simulink model "UAV"  (R2025b)
settings: Solver=ode3  StartTime=0.0  StopTime=inf  FixedStep=Sim.Ts_fisica  RelTol=1e-3
PostLoadFcn:
  | Init
InitFcn:
  | Init
model workspace (MAT data in the model file):
  Mass = 1
undefined symbols (not defined in the file): DiscIntNeverNeededParam, Drone, DWORK0, DWORK1, DWORK10, DWORK11, DWORK12, DWORK13, DWORK14, DWORK15, DWORK16, DWORK17, DWORK18, DWORK19, DWORK2, DWORK20, DWORK21, DWORK22, DWORK23, DWORK24, DWORK3, DWORK4, DWORK5, DWORK6, DWORK7, DWORK8, DWORK9, F, Light, MIL, Sim
libraries: simulink x35, slpidlib x11, vrlib x4, aerolibwind2 x2, sim3dlib x2, uavsim3dlib x2
(part 3 of 8)

== system UAV/untitledPanel1 ==
  Knob : KnobBlock  Tag=HiddenForWebPanel  PanelInfo="{\"height\":258,\"left\":614,\"panelId\":\"panelId-871049d7-78ac-4d7f-b4f9-794c823d572e\",\"top\":77,\"type\":\"panelChild\",\"version\":\"2019b\",\"width\":247,\"zIndex\":1500002}"  LabelPosition=Hide
  Knob1 : KnobBlock  Tag=HiddenForWebPanel  PanelInfo="{\"height\":258,\"left\":52,\"panelId\":\"panelId-871049d7-78ac-4d7f-b4f9-794c823d572e\",\"top\":77,\"type\":\"panelChild\",\"version\":\"2019b\",\"width\":247,\"zIndex\":1500006}"  LabelPosition=Hide  ScaleMax=15  TickInterval=1
  Knob2 : KnobBlock  Tag=HiddenForWebPanel  PanelInfo="{\"height\":258,\"left\":333,\"panelId\":\"panelId-871049d7-78ac-4d7f-b4f9-794c823d572e\",\"top\":77,\"type\":\"panelChild\",\"version\":\"2019b\",\"width\":247,\"zIndex\":1500004}"  LabelPosition=Hide  ScaleMax=360  TickInterval=45
  panelInfo : PanelWebBlock  Tag=HiddenForWebPanel  PanelInfo="{\"compacted\":false,\"height\":451,\"isActiveTab\":true,\"labels\":{\"label2380146012\":{\"deleted\":false,\"left\":81,\"settings\":{\"backgroundColor\":\"rgba(0, 0, 0, 0)\",\"bold\":true,\"font\":\"Arial\",\"fontColor\":\"#ffffff\",\"fontSize\":1.43,\"italicized\":false,\"underlined\":false},\"text\":\"WIND SPEED (m\\/s)\",\"top\":348},\"label7636309277\":{\"deleted\":false,\"left\":645,\"settings\":{\"backgroundColor\":\"rgba(0, 0, 0, 0)\",\"bold\":true,\"font\":\"Arial\",\"fontColor\":\"#ffffff\",\"fontSize\":1.38,\"italicized\":false,\"underlined\":false},\"text\":\"TURBULENCE (%)\",\"top\":351},\"label8670578771\":{\"deleted\":false,\"left\":355,\"settings\":{\"backgroundColor\":\"rgba(0, 0, 0, 0)\",\"bold\":true,\"font\":\"Arial\",\"fontColor\":\"#ffffff\",\"fontSize\":1.38,\"italicized\":false,\"underlined\":false},\"text\":\"WIND DIRECTION (°)\",\"top\":352}},\"left\":111,\"name\":\"Wind Panel\",\"panelId\":\"panelId-871049d7-78ac-4d7f-b4f9-794c823d572e\",\"popoutData\":{\"height\":547,\"left\":-1074,\"maximized\":false,\"top\":948,\"width\":926},\"popoutMode\":\"window\",\"tabIndex\":0,\"tabbedSetId\":\"tabbedSet2805598178\",\"top\":162,\"type\":\"panel\",\"version\":\"2019b\",\"visible\":true,\"width\":914,\"zIndex\":1500004}"  PanelSnapshot=<binary blob, 836232 chars, not shown>  PanelBackground=data:image/jpeg;base64,/9j/4AAQSkZJRgABAQEASABIAAD/4QAC/9sAhAAIBgYHBgUIBwcHCQkICgwUDQwLCwwZEhMPFB0aHx4dGhwcICQuJyAiLCMcHCg3KSwwMTQ0NB8nOT04MjwuMzQyAQkJCQwLDBgNDRgyIRwhMjIyMjIyMjIyMjIyMjIyMjIyMjIyMjIyMjIyMjIyMjIyMjIyMjIyMjIyMjIyMjIyMjL/wgARCAK8BOEDASIAAhEBAxEB/8QALwAAAwEBAQEBAAAAAAAAAAAAAgMEBQEABgcBAQEBAAAAAAAAAAAAAAAAAAABAv/aAAwDAQACEAMQAAAA+eDSHeM9jvAkiUsXM8YfKFVNf4xG3Yx9F75beC0s4I2dTDsW9DDIl3JSIaJ6usy6jXXHfGfPow2EebSc ...(+177280 chars)
